simulink model "BrakeboxVCU_v1"  (R2019b)
settings: Solver=VariableStepAuto  StartTime=0.0  StopTime=10.0  RelTol=1e-3

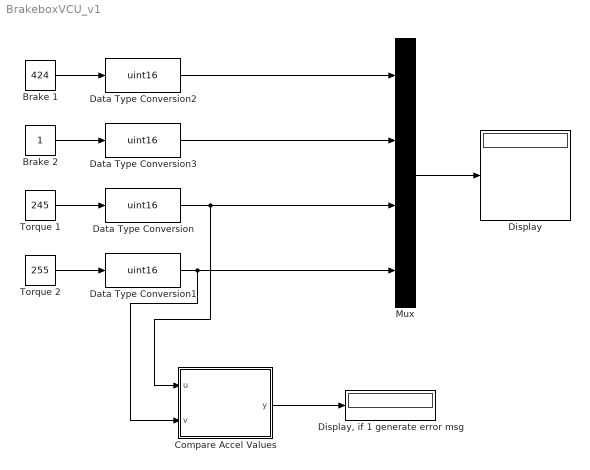
== system BrakeboxVCU_v1 ==
  Brake 1 : Constant  Value=424
  Brake 2 : Constant
  Compare Accel Values : MATLAB Function  TreatAsAtomicUnit=on
  Data Type Conversion{,1..3} (4 alike) : DataTypeConversion  OutDataTypeStr=uint16
  Display : Display
  "Display, if 1 generate error msg" : Display
  Mux : Mux
  Torque 1 : Constant  Value=245
  Torque 2 : Constant  Value=255
  wires:
  Compare Accel Values/1(y) -> "Display, if 1 generate error msg"/1
  Torque 1/1 -> Data Type Conversion/1
  Data Type Conversion/1 -> Compare Accel Values/1(u), Mux/3
  Torque 2/1 -> Data Type Conversion1/1
  Data Type Conversion1/1 -> Compare Accel Values/2(v), Mux/4
  Brake 2/1 -> Data Type Conversion3/1
  Brake 1/1 -> Data Type Conversion2/1
  Data Type Conversion3/1 -> Mux/2
  Data Type Conversion2/1 -> Mux/1
  Mux/1 -> Display/1

== matlab function BrakeboxVCU_v1/Compare Accel Values ==
  data: u input; y output; v input
function y = accelcompare(u, v)
% Checks if there is 10% difference or greater and returns 1 if true

y = (abs(u-v)/max(u,v)) >= 0.1;


end
